simulink model "NetraAI_DigitalTwin_V6_RecaptureLoop"  (Simulink 8.3)
settings: Solver=VariableStepDiscrete  StartTime=0.0  StopTime=28800  MaxStep=1  RelTol=1e-3
Description:
  | ANEYE / NetraAI Digital Twin V6. Primary and recapture acquisition traffic are merged using a SimEvents Path Combiner. Route-5 cases consume recapture preparation, a second fundus capture and a second AI pass. Recapture cases exit after the second AI pass; post-recapture clinical outcome is not inferred.
settings Model: Creator=kaustav  LastModifiedBy=kaustav
settings DataIOCC: SignalLoggingSaveFormat=Dataset
settings DebuggingCC: UnderspecifiedInitializationDetection=Simplified  StateNameClashWarn=none
settings GRTTargetCC: CombineOutputUpdateFcns=on  GRTInterface=off

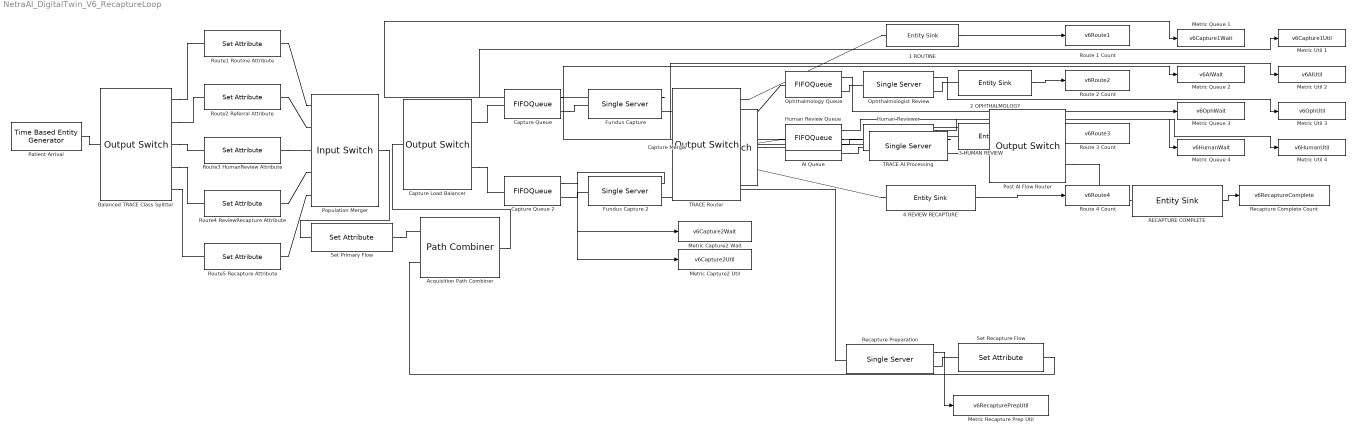
== system NetraAI_DigitalTwin_V6_RecaptureLoop ==
  1 ROUTINE : EntitySink  StatNumberArrived=on
  2 OPHTHALMOLOGY : EntitySink  StatNumberArrived=on
  3 HUMAN REVIEW : EntitySink  StatNumberArrived=on
  4 REVIEW RECAPTURE : EntitySink  StatNumberArrived=on
  AI Queue : FIFOQueue  Capacity=1000  StatAverageWait=on
      settings: OutputPortMap=o2
  Acquisition Path Combiner : PathCombiner  NumberInputPorts=2
  Balanced TRACE Class Splitter : OutputSwitch  NumberOutputPorts=5  SwitchingCriterion=Round robin
  Capture Load Balancer : OutputSwitch  NumberOutputPorts=2  SwitchingCriterion=Round robin
  Capture Merger : InputSwitch  NumberInputPorts=2
  Capture Queue : FIFOQueue  Capacity=1000  StatAverageWait=on
      settings: OutputPortMap=o2
  Capture Queue 2 : FIFOQueue  Capacity=1000  StatAverageWait=on
      settings: OutputPortMap=o2
  Fundus Capture : SingleServer  ServiceTime=120  StatUtilization=on
      settings: OutputPortMap=o5
  Fundus Capture 2 : SingleServer  ServiceTime=120  StatUtilization=on
      settings: OutputPortMap=o5
  Human Review Queue : FIFOQueue  Capacity=1000  StatAverageWait=on
      settings: OutputPortMap=o2
  Human Reviewer : SingleServer  ServiceTime=45  StatUtilization=on
      settings: OutputPortMap=o5
  Metric Capture2 Util : ToWorkspace  VariableName=v6Capture2Util  SampleTime=-1
  Metric Capture2 Wait : ToWorkspace  VariableName=v6Capture2Wait  SampleTime=-1
  Metric Queue 1 : ToWorkspace  VariableName=v6Capture1Wait  SampleTime=-1
  Metric Queue 2 : ToWorkspace  VariableName=v6AIWait  SampleTime=-1
  Metric Queue 3 : ToWorkspace  VariableName=v6OphWait  SampleTime=-1
  Metric Queue 4 : ToWorkspace  VariableName=v6HumanWait  SampleTime=-1
  Metric Recapture Prep Util : ToWorkspace  VariableName=v6RecapturePrepUtil  SampleTime=-1
  Metric Util 1 : ToWorkspace  VariableName=v6Capture1Util  SampleTime=-1
  Metric Util 2 : ToWorkspace  VariableName=v6AIUtil  SampleTime=-1
  Metric Util 3 : ToWorkspace  VariableName=v6OphUtil  SampleTime=-1
  Metric Util 4 : ToWorkspace  VariableName=v6HumanUtil  SampleTime=-1
  Ophthalmologist Review : SingleServer  ServiceTime=30  StatUtilization=on
      settings: OutputPortMap=o5
  Ophthalmology Queue : FIFOQueue  Capacity=1000  StatAverageWait=on
      settings: OutputPortMap=o2
  Patient Arrival : TimeBasedEntityGenerator  Period=86.4
  Population Merger : InputSwitch  NumberInputPorts=5
  Post AI Flow Router : OutputSwitch  NumberOutputPorts=2  SwitchingCriterion=From attribute  AttributeName=flowType
  RECAPTURE COMPLETE : EntitySink  StatNumberArrived=on
  Recapture Complete Count : ToWorkspace  VariableName=v6RecaptureComplete  SampleTime=-1
  Recapture Preparation : SingleServer  ServiceTime=20  StatUtilization=on
      settings: OutputPortMap=o5
  Route 1 Count : ToWorkspace  VariableName=v6Route1  SampleTime=-1
  Route 2 Count : ToWorkspace  VariableName=v6Route2  SampleTime=-1
  Route 3 Count : ToWorkspace  VariableName=v6Route3  SampleTime=-1
  Route 4 Count : ToWorkspace  VariableName=v6Route4  SampleTime=-1
  Route1 Routine Attribute : SetAttribute  AttributeName=routeCode  EvaluatedAttributeValue={ 1}
  Route2 Referral Attribute : SetAttribute  AttributeName=routeCode  AttributeValue=2  EvaluatedAttributeValue={ 2}
  Route3 HumanReview Attribute : SetAttribute  AttributeName=routeCode  AttributeValue=3  EvaluatedAttributeValue={ 3}
  Route4 ReviewRecapture Attribute : SetAttribute  AttributeName=routeCode  AttributeValue=4  EvaluatedAttributeValue={ 4}
  Route5 Recapture Attribute : SetAttribute  AttributeName=routeCode  AttributeValue=5  EvaluatedAttributeValue={ 5}
  Set Primary Flow : SetAttribute  AttributeName=flowType  EvaluatedAttributeValue={ 1}
  Set Recapture Flow : SetAttribute  AttributeName=flowType  AttributeValue=2  EvaluatedAttributeValue={ 2}
  TRACE AI Processing : SingleServer  ServiceTime=8.67151  StatUtilization=on
      settings: OutputPortMap=o5
  TRACE Router : OutputSwitch  NumberOutputPorts=5  SwitchingCriterion=From attribute  AttributeName=routeCode
  wires:
  1 ROUTINE/1 -> Route 1 Count/1
  2 OPHTHALMOLOGY/1 -> Route 2 Count/1
  3 HUMAN REVIEW/1 -> Route 3 Count/1
  4 REVIEW RECAPTURE/1 -> Route 4 Count/1
  Capture Queue/1 -> Metric Queue 1/1
  AI Queue/1 -> Metric Queue 2/1
  Ophthalmology Queue/1 -> Metric Queue 3/1
  Human Review Queue/1 -> Metric Queue 4/1
  Fundus Capture/1 -> Metric Util 1/1
  TRACE AI Processing/1 -> Metric Util 2/1
  Ophthalmologist Review/1 -> Metric Util 3/1
  Human Reviewer/1 -> Metric Util 4/1
  Capture Queue 2/1 -> Metric Capture2 Wait/1
  Fundus Capture 2/1 -> Metric Capture2 Util/1
  RECAPTURE COMPLETE/1 -> Recapture Complete Count/1
  Recapture Preparation/1 -> Metric Recapture Prep Util/1
  connections:
  Route1 Routine Attribute/RConn1 -- Population Merger/LConn1
  Route2 Referral Attribute/RConn1 -- Population Merger/LConn2
  Route3 HumanReview Attribute/RConn1 -- Population Merger/LConn3
  Route4 ReviewRecapture Attribute/RConn1 -- Population Merger/LConn4
  Route5 Recapture Attribute/RConn1 -- Population Merger/LConn5
  TRACE Router/RConn1 -- 1 ROUTINE/LConn1
  TRACE Router/RConn2 -- Ophthalmology Queue/LConn1
  Ophthalmology Queue/RConn1 -- Ophthalmologist Review/LConn1
  Ophthalmologist Review/RConn1 -- 2 OPHTHALMOLOGY/LConn1
  TRACE Router/RConn3 -- Human Review Queue/LConn1
  Human Review Queue/RConn1 -- Human Reviewer/LConn1
  Human Reviewer/RConn1 -- 3 HUMAN REVIEW/LConn1
  TRACE Router/RConn4 -- 4 REVIEW RECAPTURE/LConn1
  Patient Arrival/RConn1 -- Balanced TRACE Class Splitter/LConn1
  Balanced TRACE Class Splitter/RConn1 -- Route1 Routine Attribute/LConn1
  Balanced TRACE Class Splitter/RConn2 -- Route2 Referral Attribute/LConn1
  Balanced TRACE Class Splitter/RConn3 -- Route3 HumanReview Attribute/LConn1
  Balanced TRACE Class Splitter/RConn4 -- Route4 ReviewRecapture Attribute/LConn1
  Balanced TRACE Class Splitter/RConn5 -- Route5 Recapture Attribute/LConn1
  Population Merger/RConn1 -- Set Primary Flow/LConn1
  Set Primary Flow/RConn1 -- Acquisition Path Combiner/LConn1
  Acquisition Path Combiner/RConn1 -- Capture Load Balancer/LConn1
  Capture Load Balancer/RConn1 -- Capture Queue/LConn1
  Capture Load Balancer/RConn2 -- Capture Queue 2/LConn1
  Capture Queue/RConn1 -- Fundus Capture/LConn1
  Capture Queue 2/RConn1 -- Fundus Capture 2/LConn1
  Fundus Capture/RConn1 -- Capture Merger/LConn1
  Fundus Capture 2/RConn1 -- Capture Merger/LConn2
  Capture Merger/RConn1 -- AI Queue/LConn1
  AI Queue/RConn1 -- TRACE AI Processing/LConn1
  TRACE AI Processing/RConn1 -- Post AI Flow Router/LConn1
  Post AI Flow Router/RConn1 -- TRACE Router/LConn1
  Post AI Flow Router/RConn2 -- RECAPTURE COMPLETE/LConn1
  TRACE Router/RConn5 -- Recapture Preparation/LConn1
  Recapture Preparation/RConn1 -- Set Recapture Flow/LConn1
  Set Recapture Flow/RConn1 -- Acquisition Path Combiner/LConn2
